simulink subsystem "SensorSonido"  (R2023b)
settings: Solver=VariableStepAuto  StartTime=0.0  StopTime=10.0  RelTol=1e-3
libraries: arduinolib x2
settings Model: Creator=TESTER  LastModifiedBy=TESTER

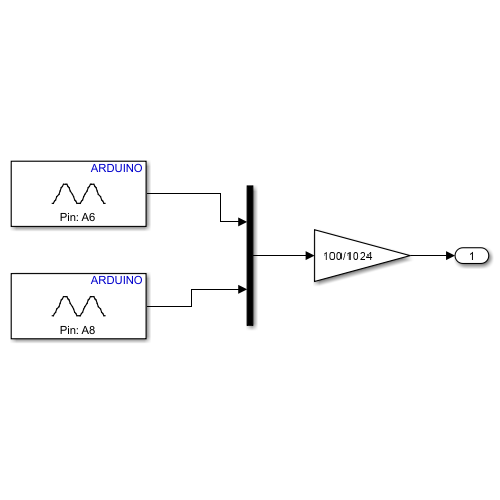
[thumbnail: Simulink's stored preview of the top-level diagram]
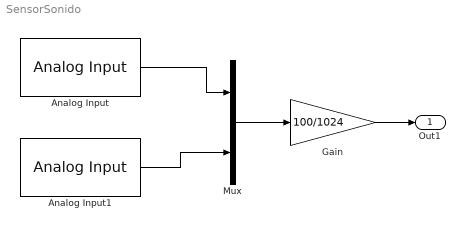
== system SensorSonido ==
  Analog Input : arduinolib/Analog Input  pinNumber=6  ReadResultsOnly=off  ConversionTriggerSource=Software  ExternalTriggerType=uint32( 0 )  OutputDataType=uint16  EnableConversionCompleteNotify=off  EnableOuputStatus=off  SampleTime=-1  blockPlatform=arduino
  Analog Input1 : arduinolib/Analog Input  pinNumber=8  ReadResultsOnly=off  ConversionTriggerSource=Software  ExternalTriggerType=uint32( 0 )  OutputDataType=uint16  EnableConversionCompleteNotify=off  EnableOuputStatus=off  SampleTime=-1  blockPlatform=arduino
  Gain : Gain  Gain=100/1024
  Mux : Mux  Inputs=2
  Out1 : Outport
  wires:
  Mux/1 -> Gain/1
  Gain/1 -> Out1/1
  Analog Input/1 -> Mux/1
  Analog Input1/1 -> Mux/2
